simulink model "TPEtape2simulink"  (R2025b)
settings: Solver=VariableStepAuto  StartTime=0.0  StopTime=70000  RelTol=1e-3
values from neighbouring files (symbols this model uses):
  K2 = 5 * 10^(-3)    (= 0.005)    [Partie1TPauto.m]    (also in Partie2TPauto.m; Partie3TPauto.m)
  Kp = 10    [Partie2TPauto.m]
  newKp = 1    [Partie2TPauto.m]
libraries: cstblocks x4
settings Model: Creator=dayan  LastModifiedBy=dayan

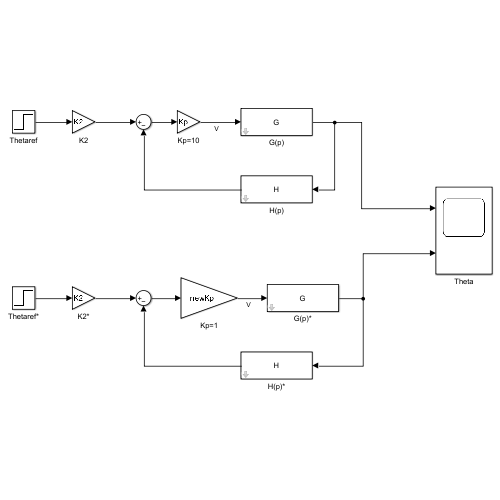
[thumbnail: Simulink's stored preview of the top-level diagram]
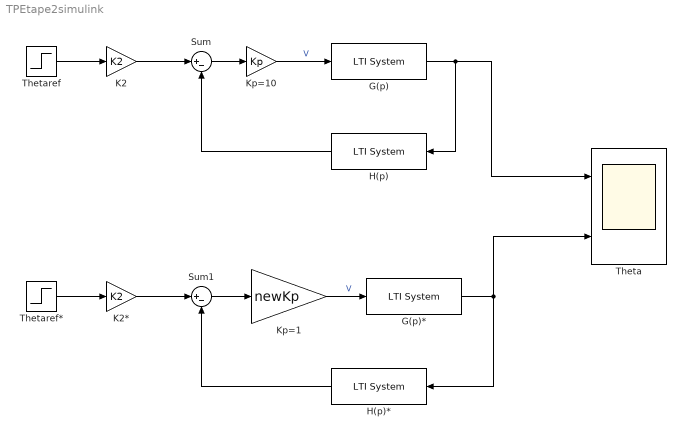
== system TPEtape2simulink ==
  G(p) : cstblocks/LTI System  sys=G  IC=[]  PadeOrder=0
  G(p)* : cstblocks/LTI System  sys=G  IC=[]  PadeOrder=0
  H(p) : cstblocks/LTI System  sys=H  IC=[]  PadeOrder=0
  H(p)* : cstblocks/LTI System  sys=H  IC=[]  PadeOrder=0
  K2 : Gain  Gain=K2
  K2* : Gain  Gain=K2
  Kp=1 : Gain  Gain=newKp
  Kp=10 : Gain  Gain=Kp
  Sum : Sum  Inputs=|+-
  Sum1 : Sum  Inputs=|+-
  Theta : Scope  NumInputPorts=2
      settings: ActiveDisplayYMinimum=-195.8758249521166  ActiveDisplayYMaximum=1762.8824245690498
  Thetaref : Step  Time=0  After=1200  SampleTime=0
  Thetaref* : Step  Time=0  After=1200  SampleTime=0
  wires:
  Thetaref/1 -> K2/1
  K2/1 -> Sum/1
  Sum/1 -> Kp=10/1
  Kp=10/1 -> G(p)/1  "V"
  G(p)/1 -> Theta/1, H(p)/1
  H(p)/1 -> Sum/2
  G(p)*/1 -> H(p)*/1, Theta/2
  Kp=1/1 -> G(p)*/1  "V"
  Thetaref*/1 -> K2*/1
  H(p)*/1 -> Sum1/2
  Sum1/1 -> Kp=1/1
  K2*/1 -> Sum1/1
